simulink model "BrushlessDCMotor"  (R2020a)
settings: Solver=VariableStepAuto  StartTime=0.0  StopTime=10.0  RelTol=1e-3
undefined symbols (not defined in the file or in its folder): PM
libraries: spsPMSynchronousMachineModel x3, simulink x1
settings Model: Creator=Sony  LastModifiedBy=Sony

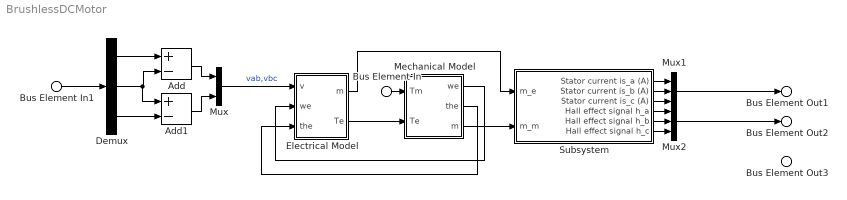
== system BrushlessDCMotor ==
  Bus Element In1 : Inport  PortName=AC Stator Voltages VABC
  Bus Element In : Inport  Port=2  PortName=Tm
  Add : Sum  Inputs=+-
  Add1 : Sum  Inputs=+-
  Demux : Demux  Outputs=3
  Electrical Model : Subsystem
  Mechanical Model : Subsystem
  Mux : Mux  Inputs=2
  Mux1 : Mux  Inputs=3
  Mux2 : Mux  Inputs=3
  Subsystem : Subsystem
  Bus Element Out1 : Outport  PortName=Stator Phase Currents IABC
  Bus Element Out2 : Outport  Port=2  PortName=HALL Sensor Signals HABC
  Bus Element Out3 : Outport  Port=3  PortName=Temperature
  wires:
  Subsystem/5(Hall effect signal h_b) -> Mux2/2
  Subsystem/4(Hall effect signal h_a) -> Mux2/1
  Add1/1 -> Mux/2
  Subsystem/3(Stator current is_c (A)) -> Mux1/3
  Electrical Model/1(m) -> Subsystem/1(m_e)
  Subsystem/2(Stator current is_b (A)) -> Mux1/2
  Bus Element In/1 -> Mechanical Model/1(Tm)
  Mechanical Model/1(we) -> Electrical Model/2(we)
  Electrical Model/2(Te) -> Mechanical Model/2(Te)
  Mechanical Model/3(m) -> Subsystem/2(m_m)
  Mechanical Model/2(the) -> Electrical Model/3(the)
  Demux/3 -> Add1/2
  Add/1 -> Mux/1
  Subsystem/1(Stator current is_a (A)) -> Mux1/1
  Mux1/1 -> Bus Element Out1/1
  Demux/2 -> Add1/1, Add/2
  Subsystem/6(Hall effect signal h_c) -> Mux2/3
  Demux/1 -> Add/1
  Mux/1 -> Electrical Model/1(v)  "vab,vbc"
  Mux2/1 -> Bus Element Out2/1
  Bus Element In1/1 -> Demux/1

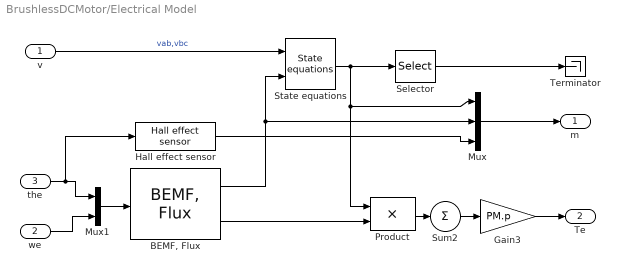
== system BrushlessDCMotor/Electrical Model ==
  v : Inport
  we : Inport  Port=2
  the : Inport  Port=3
  "BEMF, Flux" : spsPMSynchronousMachineModel/Continuous Trapezoidal/BEMF, Flux
      settings: SourceProductBaseCode=PS
  Gain3 : Gain  Gain=PM.p  SaturateOnIntegerOverflow=on  OutDataTypeStr=Inherit: Same as input  ParamDataTypeStr=Inherit: Same as input
  Hall effect sensor : spsPMSynchronousMachineModel/Continuous Trapezoidal/Hall effect sensor
      settings: SourceProductBaseCode=PS
  Mux : Mux  Inputs=3
  Mux1 : Mux  Inputs=2
  Product : Product  SaturateOnIntegerOverflow=on  OutDataTypeStr=Inherit: Same as first input
  Selector : Selector  InputPortWidth=3  IndexOptions=Index vector (dialog)  Indices=1:2  OutputSizes=1
  State equations : spsPMSynchronousMachineModel/Continuous Trapezoidal/State equations
      settings: SourceProductBaseCode=PS
  Sum2 : Sum  Inputs=+  SaturateOnIntegerOverflow=on
  Terminator : Terminator
  m : Outport  InitialOutput=0
  Te : Outport  Port=2  InitialOutput=0
  wires:
  "BEMF, Flux"/1 -> Mux/2, State equations/2
  Gain3/1 -> Te/1
  Selector/1 -> Terminator/1
  we/1 -> Mux1/2
  Mux/1 -> m/1
  Hall effect sensor/1 -> Mux/3
  Product/1 -> Sum2/1
  Sum2/1 -> Gain3/1
  the/1 -> Hall effect sensor/1, Mux1/1
  State equations/1 -> Mux/1, Product/1, Selector/1
  Mux1/1 -> "BEMF, Flux"/1
  "BEMF, Flux"/2 -> Product/2
  v/1 -> State equations/1  "vab,vbc"

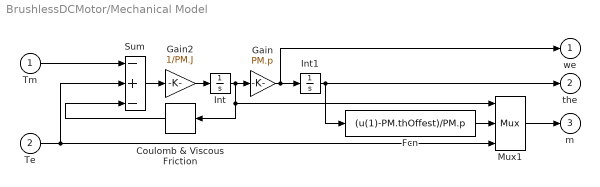
== system BrushlessDCMotor/Mechanical Model ==
  Tm : Inport
  Te : Inport  Port=2
  Coulomb & Viscous Friction : simulink/Discontinuities/Coulomb & Viscous Friction  offset=PM.Tf  gain=PM.F
  Fcn : Fcn  Expr=(u(1)-PM.thOffest)/PM.p
  Gain : Gain  Gain=PM.p  SaturateOnIntegerOverflow=on  OutDataTypeStr=Inherit: Same as input  ParamDataTypeStr=Inherit: Same as input
  Gain2 : Gain  Gain=1/PM.J  SaturateOnIntegerOverflow=on  OutDataTypeStr=Inherit: Same as input  ParamDataTypeStr=Inherit: Same as input
  Int : Integrator  InitialCondition=PM.wmo
  Int1 : Integrator  InitialCondition=PM.tho+PM.thOffest
  Mux1 : Mux  Inputs=3
  Sum : Sum  Inputs=-+-  InputSameDT=on  SaturateOnIntegerOverflow=on  OutDataTypeStr=Inherit: Same as first input
  we : Outport  InitialOutput=0
  the : Outport  Port=2  InitialOutput=0
  m : Outport  Port=3  InitialOutput=0
  wires:
  Fcn/1 -> Mux1/2
  Coulomb & Viscous Friction/1 -> Sum/3
  Mux1/1 -> m/1
  Tm/1 -> Sum/1
  Int1/1 -> the/1, Fcn/1
  Gain2/1 -> Int/1
  Gain/1 -> we/1, Int1/1
  Sum/1 -> Gain2/1
  Int/1 -> Gain/1, Coulomb & Viscous Friction/1, Mux1/1
  Te/1 -> Sum/2, Mux1/3

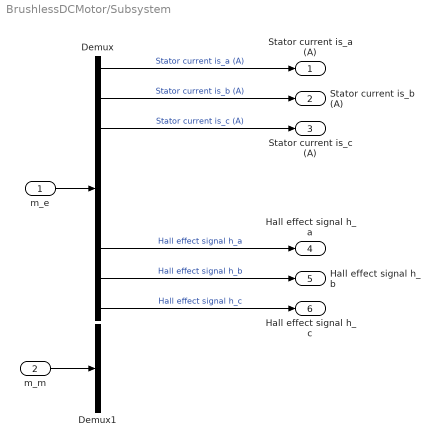
== system BrushlessDCMotor/Subsystem ==
  m_e : Inport
  m_m : Inport  Port=2
  Demux : Demux  Outputs=[1,1,1,1,1,1,1,1,1]
  Demux1 : Demux  Outputs=[1,1,1]
  Stator current is_a (A) : Outport
  Stator current is_b (A) : Outport  Port=2
  Stator current is_c (A) : Outport  Port=3
  Hall effect signal h_a : Outport  Port=4
  Hall effect signal h_b : Outport  Port=5
  Hall effect signal h_c : Outport  Port=6
  wires:
  m_m/1 -> Demux1/1
  Demux/3 -> Stator current is_c (A)/1  "Stator current is_c (A)"
  Demux/1 -> Stator current is_a (A)/1  "Stator current is_a (A)"
  Demux/2 -> Stator current is_b (A)/1  "Stator current is_b (A)"
  Demux/9 -> Hall effect signal h_c/1  "Hall effect signal h_c"
  Demux/8 -> Hall effect signal h_b/1  "Hall effect signal h_b"
  Demux/7 -> Hall effect signal h_a/1  "Hall effect signal h_a"
  m_e/1 -> Demux/1
